simulink model "BasicAudio_Target"  (R2022b)
settings: Solver=FixedStepDiscrete  StartTime=0.0  StopTime=1  RelTol=1e-3  EnableMultiTasking=on
InitFcn:
  | % Initialize model
  | run([ ModelRootName() 'Init.m' ]);
  | 
  | % load library data
  | GainLibrary_data;
  | % Load saved values from partition process
  | TOP_Mask.LoadMapFromFile(bdroot)
model workspace (MAT data in the model file):
  PreampVolumeTable_Idx : Simulink.Signal (value not decoded)
  Range : Simulink.Signal (value not decoded)
  Table_Idx : Simulink.Signal (value not decoded)
undefined symbols (not defined in the file or in its folder): ModelCfg, RgainBusUtil
libraries: TOP x27, HandyTextFile x14, FeaturePath x7, SetDsm x6, RTC x5, AudioStats x3, CapturedConstLib x3, EdgePorts x2, MuteRamperBtc x1, RgainyBtc x1, simulink_need_slupdate x1, dspsrcs4 x1
(part 5 of 5)

== matlab function BasicAudio_Target/BasicAudio/Bass/Tone/InnerLink/ramp parameters ==
  data: data input; ramptime output; rampTimeRTC input; rampRateRTC input; rampRate output; rampRateBounds parameter; rampTimeBounds parameter
  events: trigger input FUNCTION_CALL_EVENT
function [ramptime, rampRate]  = ramp_parameters( data, rampTimeRTC, rampRateRTC,... % inputs
    rampRateBounds, rampTimeBounds) % parameters

%#codegen
    % Ramp time mentioned in the RTC message gets priority over the tune
    % variable. Boundary conditions are also included based on BDSP values.
    % If neither ramp time nor rate are given in the RTC message (i.e. both
    % = 0), then the ramp time in the Tune variable is taken as the default
    % value for that message.
    
    ramptime = single(data);
    rampRate = single(0); 
    
    if (rampRateRTC)
        rampRate = single(rampRateRTC);
        rampRate = max(rampRateBounds(1), rampRate);
        rampRate = min(rampRateBounds(2), rampRate);
    end
    if (rampTimeRTC)
        ramptime = single(rampTimeRTC);
    end
    ramptime = max(rampTimeBounds(1), ramptime);
    ramptime = min(rampTimeBounds(2), ramptime);
end

== matlab function BasicAudio_Target/BasicAudio/Bass/Tone/InnerLink/check done ==
  data: done output; Rampers data_store_memory
  events: trigger input FUNCTION_CALL_EVENT
function done  = fcn
%#codegen

global Rampers;

% Checking whether the frameCounts are exactly equal to 0 was leading to
% unpredictable behavior. Therefore, we now check whether or not the 
% frameCounts are less-than/equal-to 0.
% See SAMPLERATE-1196 & SAMPLERATE-1205 for more details. 
done = (Rampers(1).frameCount <= 0) && (Rampers(2).frameCount <= 0);

== matlab function BasicAudio_Target/BasicAudio/Bass/Tone/InnerLink/index to linear ==
  data: linearGain output; scale input; offset input; index input
  events: trigger input FUNCTION_CALL_EVENT
function linearGain = compute_gain(scale,offset,index)
%#codegen

% The midrange curve is configured as a piecewise linear plot, with
% configurable values of the maximum boost ('maxB') and maximum cut ('maxC')
% in dB. 
%    dB ^
%       |
% maxB  ----------/
%       |        /
%       |       /
%  0    ------|---|----> index
%       |   /128  255
%       |  /
% maxC  --/
%       |
% Hence, for any given index, the gain is calculated as a value in 
% between 0 and 1 for boost and 0 and -1 for cut. This will later be
% multiplied with the maxB or maxC to get the actual gain value. 
% (y - y1) / (x - x1) = (y1 - y2) / (x1 - x2)
% (y - 0) / (x - 128) = (0 - 1) / (128 - 255)
%                   y = (x - 128)/127
% 'offset' represents the center point between boost and cut (i.e. 128) and
% 'scale' represents how many intervals are available for boost/cut (i.e. 127)

% Apply the tuning calibration
floatIndex = single(index);
linearGain = single((floatIndex - offset) / scale);

% Ensure the result is between -1 and 1
linearGain = min(linearGain, 1);
linearGain = max(linearGain, -1);

== matlab function BasicAudio_Target/BasicAudio/Bass/Tone/InnerLink/tone ==
  data: audioOut output; boost_coeffs input; cut_coeffs input; audioIn input; Rampers data_store_memory; gain output; Freeze data_store_memory; Phase data_store_memory
function [audioOut,gain] ...
    = toneProcess(boost_coeffs, cut_coeffs, audioIn)...    % inputs % parameters
  
%#codegen

% Data Store objects (registered in "Edit Data" dialog
global Rampers;
global Freeze;
global Phase;

% Keep memory for the filter persistent from frame to frame
persistent toneFilterStates;

% figure out the frame size and channel count
[frame_size, channel_count] = size(audioIn);

if (isempty(toneFilterStates))
    toneFilterStates = zeros(1,channel_count,'single');
end


% set the size and datatype of the output buffer
audioOut = coder.nullcopy(audioIn);

ramper = Phase;
ramperCount = numel(Rampers);

if (Freeze == false)
    if (Rampers(ramper).frameCount == 0)
        % The current ramper is finished. Is there another one?
        if (ramper < ramperCount && Rampers(ramper+1).frameCount > 0)
            % Yes - move on to the next phase
            ramper = ramper + 1;
            Phase = ramper;
            k = Rampers(ramper).rampCoeff;
            gain = Rampers(ramper).currentGain;
            Rampers(ramper).frameCount = Rampers(ramper).frameCount - 1;
        else
            %  Stop ramping and SNAP to the target
            k = single(1);
            gain = Rampers(ramper).targetGain;
            % Update completion flag
         end
    else
        % The ramp is *NOT* frozen or done: gain is moving
        k = Rampers(ramper).rampCoeff;
        gain = Rampers(ramper).currentGain;
        Rampers(ramper).frameCount = Rampers(ramper).frameCount - 1;
    end
else
    % Frozen. Stay at current gain
    k = single(1);
    gain = Rampers(ramper).currentGain;
end

% Apply the tone filter
if (gain < 1)
    % Cut
    bCoeffs = cut_coeffs(1:2);
    aCoeffs = cut_coeffs(3);
else
    % Boost
    bCoeffs = boost_coeffs(1:2);
    aCoeffs = boost_coeffs(3);
end

% [filtered,toneFilterStates] = filter(bCoeffs, aCoeffs, audioIn, toneFilterStates);

% Loop through samples, adjusting gain and applying to channels
for n=1:frame_size
    % Update the gain and then subtract one before applying it to the
    % filtered signal. Disregarding phase shifting 
    gain = gain * k;
    filterGain = gain - 1;
    % Loop through channels adding in gain-adjusted filtered samples
    for chanIdx = 1:channel_count
        
        filterOut = (bCoeffs(1) * audioIn(n,chanIdx)) + toneFilterStates(chanIdx);
        toneFilterStates(chanIdx) = (bCoeffs(2) * audioIn(n,chanIdx)) + (aCoeffs(1) * filterOut);
        
        audioOut(n,chanIdx) = audioIn(n,chanIdx) + (filterOut * filterGain);
    end
end

Rampers(ramper).currentGain = gain;

== matlab function BasicAudio_Target/BasicAudio/Bass/Tone/InnerLink/tone control ==
  data normalized_gain_impact settings: description=This vector signal must provide a linear target gain for every ramper.
  data db_per_sec settings: description="If provided (i.e. non zero), this argument causes the \"ramp times (ms)\" input to be ignored. The block will calculate ramp times itself to ensure all gain changes happen at the db_per_sec slope provided."
  data ramp_time_ms settings: description=|
      | The rampTimes_ms signal can accept one or more ramp times. If only one time is given, it is applied to all rampers. When more than one time is given, the times are delt out to the rampers in order. If not enough times are specified to cover all the rampers, the last given time is filled in to any remaining rampers.
      | NOTE: this input signal is entirely ignored if the db_per_sec input signal is non-zero. Attach the db_per_sec input to a ground block if you want to provide ramp times via this input.
  data sample_rate_in_hertz settings: description="This input is required for control calculations to work. The \"Audio Stats\" block is a handy tool to lift this property right off an inbound audio signal and feed it to this block automatically without using workspace parameters or other constants."
  data frame_size settings: description="This input is required for control calculations to work. The \"Audio Stats\" block is a handy tool to lift this property right off an inbound audio signal and feed it to this block automatically without using workspace parameters or other constants."
  data: boost_max_db input; cut_max_db input; normalized_gain_impact input size=1; db_per_sec input; ramp_time_ms input; sample_rate_in_hertz input; frame_size input; Rampers data_store_memory; rgain_SILENT_GAIN parameter; Phase data_store_memory
  events: trigger input FUNCTION_CALL_EVENT
function control(...
    boost_max_db, cut_max_db, ... %inputs
    normalized_gain_impact, db_per_sec, ramp_time_ms, sample_rate_in_hertz, frame_size, ... % inputs % parameters
    rgain_SILENT_GAIN) %parameters

% See Control summary at the end:
global Phase;
global Rampers;

% Step 1: FREEZE the gain ramper so that we can perform calculations based
% on the current gain value. (This step now performed on canvas)

% Step 2a: IMPACT-TARGET Translate the normalized gain into a dB impact
% based on the maximum boost or cut values.
% ("-1" = maximum cut, "1" = maximum boost.)
targetIsBoost = (normalized_gain_impact >= 0);
if (targetIsBoost)
    targetImpact_db = normalized_gain_impact * boost_max_db;
    targetEffectiveGain = undb20(targetImpact_db); % 1 or greater
else
    targetImpact_db = normalized_gain_impact * cut_max_db;
    targetEffectiveGain = undb20(targetImpact_db); % less than 1
end

actualTargetGainLinear = targetEffectiveGain; 

% Step 2b: IMPACT-CURRENT Fetch the current gain from the previously
% active ramper.
currentPhase = Phase;
currentGain = Rampers(currentPhase).currentGain;
currentIsBoost = (currentGain >= 1);
currentImpact_db = db20(currentGain);

% Setup processing to continue on seamlessly while we work here
Rampers(1).currentGain = currentGain;
Phase = uint32(1); % reset phase to 1
% Now that we have both current and target impacts, find the difference
db_diff = abs(currentImpact_db - targetImpact_db);

% Step 3a: TIME- If a slope in dB/second is provided, ignore the ramp time
if (db_per_sec)
    ramp_ms = db_diff / single(db_per_sec) * 1000;
else
    ramp_ms = single(ramp_time_ms);
end
    
% Step 3b: TIME- QUANTIZE the desired ramp time to our FrameSize. 
quantum_ms = 1000 * frame_size / sample_rate_in_hertz;
numFrames = ramp_ms / quantum_ms;
numFrames = max (1, ceil(numFrames));

% Step 4a: PHASES- Determine whether ramping from current gain to target
% gain requires a unity crossing in linear gain.
isTwoPhase = (currentIsBoost ~= targetIsBoost) && ...
             (currentGain ~= 1) && ... % cannot cross if you're already there
             (targetImpact_db ~= 1);  % no crossing needed when impact already nothing
% Setup a structure to hold information about what the rampers should do
twoSingles = {single(0) single(0)};
phaseConfig = struct('frames',twoSingles,'target_linear',twoSingles,'current_linear',twoSingles);
phaseConfig = tone_control_split(numFrames,currentImpact_db,db_diff,...
    currentGain,currentIsBoost,rgain_SILENT_GAIN,targetIsBoost,...
    targetEffectiveGain,isTwoPhase,phaseConfig);

% Step 4b: PHASES- Setup rampers for both phases
for currentPhase=1:2
    if (phaseConfig(currentPhase).frames)
        ramp_ms = quantum_ms * phaseConfig(currentPhase).frames;
        factor = log(phaseConfig(currentPhase).target_linear / phaseConfig(currentPhase).current_linear);
        RampCoef = exp(factor / (sample_rate_in_hertz * ramp_ms / 1000));
    else
        RampCoef = single(1);
    end
    Rampers(currentPhase).rampCoeff   = single(RampCoef);
    Rampers(currentPhase).targetGain  = actualTargetGainLinear; % phase 1 value ignored.
    Rampers(currentPhase).currentGain = single(phaseConfig(currentPhase).current_linear);
    Rampers(currentPhase).frameCount  = int32(phaseConfig(currentPhase).frames);
end

% unfreeze the gain. (This step now performed on canvas)


end

% Nudge the gain values a bit if they are sitting right at one (aka unity).
% When a control set goes live, ensure that the current gain will move.
% If current gain is one, replace with a value very close to one. What we
% really want is a value which is on the edge of perception - not too small
% or large. If the value is too small, we'll waste some of our ramp time
% in perceived silence. If the value is too large, the audio will lurch
% into perceptability at the start of the ramp. Remember that normally we
% worry about gains of 0 -- this checks instead against 1 because filter
% gain is effective gain minuus 1.
function adjustedLinearGain = NudgeUnity(linearGain,isPositive,silentGain)
    if (isPositive)
        adjustedLinearGain = max(linearGain, 1 + silentGain);
    else
        adjustedLinearGain = min(linearGain, 1 - silentGain);
    end
end

function phaseConfig = tone_control_split(numFrames,currentImpact_db,db_diff,...
    currentGain,currentIsBoost,rgain_SILENT_GAIN,targetIsBoost,...
    targetEffectiveGain,isTwoPhase,phaseConfig)
if (isTwoPhase)
    % Both boost and cut phases will be required to get where we are going.
    % Make sure we have at least two frames to work with:
    numFrames = max (2, round(numFrames));
    
    % Divide up our ramp time into pieces for each phase to use
    phase1Frames = ceil(numFrames * abs(currentImpact_db) / db_diff);
    phase2Frames = numFrames - phase1Frames;
    
    % Make sure phase 2 has at least 1 frame to work with
    phase2Frames = max(1, phase2Frames);
    
    % Setup Phase 1 ramper that takes us to zero impact (i.e. unity gain)
    phaseConfig(1).current_linear   = currentGain;  % we know this is not 1
    phaseConfig(1).target_linear    = NudgeUnity(1,currentIsBoost,rgain_SILENT_GAIN);
    phaseConfig(1).frames           = phase1Frames;
    
    % Setup Phase 2 ramper that delivers us to target impact
    phaseConfig(2).current_linear   = NudgeUnity(1,targetIsBoost,rgain_SILENT_GAIN); % start quiet
    phaseConfig(2).target_linear    = targetEffectiveGain;   % we know this is not 0
    phaseConfig(2).frames           = phase2Frames;
else
    % Only one phase is needed to accomplish our goal. We are are the
    % target side of unity... but we must determine which side that is
    if (currentGain == 1)
        % One is in-between sides: use the target to determine the side
        isBoost = targetIsBoost;
    else
        % Current gain is already on one side of unity so use that
        isBoost = currentIsBoost;
    end
    phaseConfig(1).current_linear   = NudgeUnity(currentGain,isBoost,rgain_SILENT_GAIN);
    phaseConfig(1).target_linear    = NudgeUnity(targetEffectiveGain,isBoost,rgain_SILENT_GAIN);
    phaseConfig(1).frames           = numFrames;
    
    % Setup Phase 2 ramper to sit at the target gain
    phaseConfig(2).current_linear   = NudgeUnity(targetEffectiveGain,isBoost,rgain_SILENT_GAIN);
    phaseConfig(2).target_linear    = NudgeUnity(targetEffectiveGain,isBoost,rgain_SILENT_GAIN);
    phaseConfig(2).frames           = single(0);
end
end

% This routine sets up the control data that directs the operation of
% the signal processing logic. The high level design of the tone block
% involves filtering out frequency range of the signal and then mixing it
% back in. This results in a boost or a cut to the filtered frequencies. As
% such, the gain of the filtered signal equals the overall tone block's
% effective gain minus 1 for the unfiltered signal.
%
% FilterGain = EffectiveGain - 1
%                             _
%                            / \   EffectiveGain
%   >-------+-------------->| + |------------------>
%           |                \ /
%           v                 |
%      +----+---+             ^
%      |        |            / \
%      | Filter |           /   \ FilterGain
%      |        |          /gain \
%      +----+---+          +-----+
%           |                 ^
%           |                 |
%           +-----------------+
%
% Another issue of note is that crossing over from boost to cut or vice
% versa involves numerically crossing 0 in terms of the filter gain (or
% crossing 1 in terms of effective gain). When the intended impact is 0 the
% filter gain is 0... so no impact to signal because the filtered signal is
% attenuated to 0. Since filter gain changes exponentially so as to be
% linear in dB space, it is impossible to cross past 0 (from boosting to
% cutting for instance) via multiplication alone. To combat this challenge,
% this block enlists two rampers. When a single gain change involves
% crossing over the boost/cut boundary, the first ramper takes gain up yo
% the boundary and then the second ramper is set up to continue the journey
% on the other side of the boundary to ultimately reach the target impact
% gain.
%
% Inputs:
%   boost_max_db, cut_max_db: indicates maximum impact of tone impact in dB
%        which must be positive. A negative cut dB would imply a boost!
%   normalized_gain_impact : Target impact of the tone filter that must be
%        between -1 and 1. A value of "0" implies no effect, 1 and -1 are
%        maximum boost and cut respectively.
% Control Data:
%   FreezePhase(1) freezes the processing during this control operation
%   FreezePhase(2) indicates the current phase- always reset here to 1. The
%        phase indicates which of the two rampers is active. Once the first
%        ramper finishes, the second takes over (potentially to do
%        nothing if the adjustment did not require a boost/cut crossing)
%   Rampers(1) is the first phase ramper. Boost vs. cut is determined by
%        the sign of the linear current gain.
%   Rampers(2) is the second phase ramper. Boost vs. cut is determined by
%        the sign of the linear current gain.
%   *Note that the gain present in the rampers is the EFFECTIVE gain (aka
%   filter gain plus one).

% Step 4b: PHASES- Setup rampers for both phases
    % In order to have the desired ramp time, the slope must vary dependent
    % on the gain difference between target and current value.
    % Ramper's coefficient is therefore calculated as follows:
    %
    %   TargetGain = CurrentGain *( RampCoef ^ (Fs*RampTime_ms/1000) )
    %
    % therefore...
    %
    %                     log(TargetGain/CurrentGain)
    %   log(RampCoef) = ------------------------------
    %                        Fs*(RampTime_ms/1000)
    %
